simulink model "Project"  (R2021b)
settings: Solver=VariableStepAuto  StartTime=0.0  StopTime=0.02  RelTol=1e-3
model workspace (MAT data in the model file):
  a0 = [1 1 1 1 1 1 1 1 1 1]
undefined symbols (not defined in the file or in its folder): magnitude
libraries: dspstat3 x7, commrflib2 x3, commfilt2 x1
settings Model: Creator=davit  LastModifiedBy=ludovicomazzi
settings SolverCC: AlgebraicLoopSolver=TrustRegion
settings DebuggingCC: SFMachineParentedDataDiag=warning

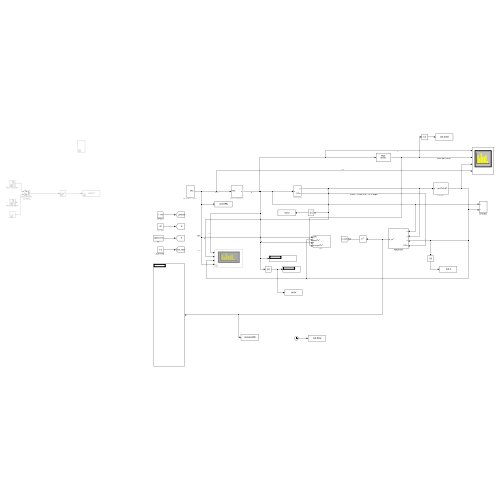
[thumbnail: Simulink's stored preview of the top-level diagram]
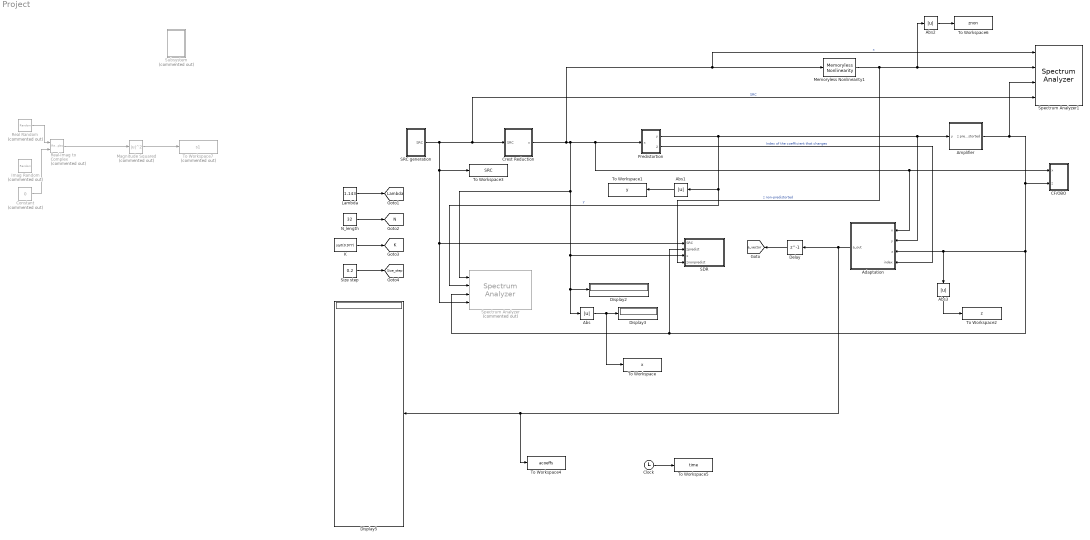
== system Project ==
  Abs{,1..3} (4 alike) : Abs
  Adaptation : Subsystem
  Amplifier : Subsystem
  CF/OBO : Subsystem
  Clock : Clock
  Constant : Constant  Commented=on  Value=0
  Crest Reduction : Subsystem
  Delay : Delay  DelayLength=1
  Display2 : Display
  Display3 : Display
  Display5 : Display
  Imag Random : RandomNumber  Commented=on  Seed=2  SampleTime=1e-7
  K : Constant  Value=sqrt(0.977)
  Lambda : Constant  Value=1.143
  Magnitude Squared : Math  Commented=on  Operator=magnitude^2  SaturateOnIntegerOverflow=on
  Memoryless Nonlinearity1 : commrflib2/Memoryless Nonlinearity  model_select=Rapp model  linGaindB=0  GindB=0  iip3=30  am2pm=10  LPwrLimAMPM=10  UPwrLimAMPM=inf  amam=[2.1587 1.1517]  ampm=[4.0033 9.1040]  x=[8.1081 1.5413 6.5202 -0.0718]  y=[4.6645 2.0965 10.88 -0.003]  p=2.5  GoutdB=0  vsat=1
      settings: SourceProductBaseCode=CM
  N_length : Constant  Value=32
  Predistortion : Subsystem
  Real Random : RandomNumber  Commented=on  Seed=1  SampleTime=1e-7
  Real-Imag to Complex : RealImagToComplex  Commented=on
  SDR : Subsystem
  SRC generation : Subsystem
  Size step : Constant  Value=0.2
  Spectrum Analyzer : SpectrumAnalyzer  Commented=on  NumInputPorts=4
  Spectrum Analyzer1 : SpectrumAnalyzer  NumInputPorts=4
  Subsystem : Subsystem  Commented=on
  To Workspace : ToWorkspace  VariableName=x  SampleTime=-1
      settings: Save2DSignal=2-D array (concatenate along first dimension)
  To Workspace1 : ToWorkspace  VariableName=y  SampleTime=-1
      settings: Save2DSignal=2-D array (concatenate along first dimension)
  To Workspace2 : ToWorkspace  VariableName=z  SampleTime=-1
      settings: Save2DSignal=2-D array (concatenate along first dimension)
  To Workspace3 : ToWorkspace  VariableName=SRC  SampleTime=-1
  To Workspace4 : ToWorkspace  VariableName=acoeffs  SampleTime=-1
      settings: Save2DSignal=2-D array (concatenate along first dimension)
  To Workspace5 : ToWorkspace  VariableName=time  SampleTime=-1
      settings: Save2DSignal=2-D array (concatenate along first dimension)
  To Workspace6 : ToWorkspace  VariableName=znon  SampleTime=-1
      settings: Save2DSignal=2-D array (concatenate along first dimension)
  To Workspace7 : ToWorkspace  Commented=on  VariableName=s1  SampleTime=-1
      settings: Save2DSignal=2-D array (concatenate along first dimension)
  tag scope: K=global, Lambda=global, N=global, Size_step=global, a_vector=global
  wires:
  SRC generation/1(SRC) -> To Workspace3/1, SDR/1(SRC), Spectrum Analyzer/4, Crest Reduction/1(SRC), Spectrum Analyzer1/4  "SRC"
  Crest Reduction/1(x) -> Abs/1, Display2/1, SDR/3(x), Spectrum Analyzer/1, Adaptation/1(x), CF/OBO/1(x), Predistortion/1(x), Spectrum Analyzer1/1, Memoryless Nonlinearity1/1  "x"
  Delay/1 -> [a_vector]
  Abs/1 -> To Workspace/1, Display3/1
  Adaptation/1(a_out) -> Delay/1, To Workspace4/1, Display5/1
  Predistortion/1(y) -> Spectrum Analyzer/2, Abs1/1, Amplifier/1(y), Adaptation/2(y)  "y"
  Predistortion/2(index) -> Adaptation/4(index)  "Index of the coefficient that changes"
  Abs1/1 -> To Workspace1/1
  Lambda/1 -> [Lambda]
  N_length/1 -> [N]
  K/1 -> [K]
  Size step/1 -> [Size_step]
  Clock/1 -> To Workspace5/1
  Memoryless Nonlinearity1/1 -> Spectrum Analyzer1/2, Abs2/1, SDR/4(znonpredist)  "z non-predistorted"
  Abs2/1 -> To Workspace6/1
  Abs3/1 -> To Workspace2/1
  Amplifier/1(z predistorted) -> Spectrum Analyzer1/3, SDR/2(zpredist), Spectrum Analyzer/3, Abs3/1, Adaptation/3(z), CF/OBO/2(z)
  Magnitude Squared/1 -> To Workspace7/1
  Real-Imag to Complex/1 -> Magnitude Squared/1
  Real Random/1 -> Real-Imag to Complex/1
  Constant/1 -> Real-Imag to Complex/2

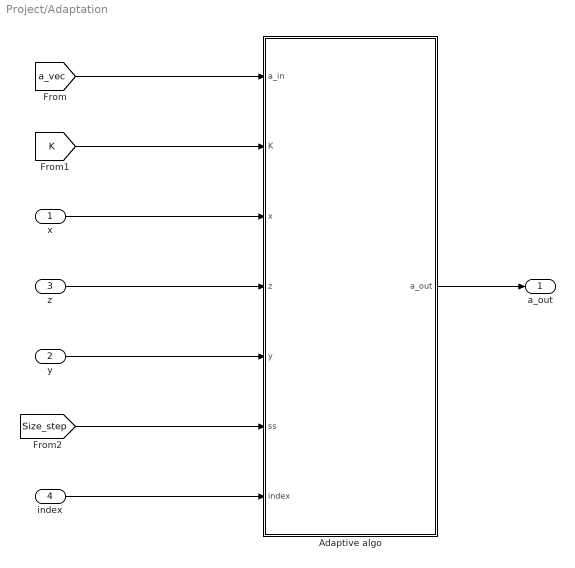
== system Project/Adaptation ==
  x : Inport
  y : Inport  Port=2
  z : Inport  Port=3
  index : Inport  Port=4
  Adaptive algo : MATLAB Function  TreatAsAtomicUnit=on
  a_out : Outport
  wires:
  y/1 -> Adaptive algo/5(y)
  index/1 -> Adaptive algo/7(index)
  z/1 -> Adaptive algo/4(z)
  Adaptive algo/1(a_out) -> a_out/1
  x/1 -> Adaptive algo/3(x)
  [K] -> Adaptive algo/2(K)
  [Size_step] -> Adaptive algo/6(ss)
  [a_vec] -> Adaptive algo/1(a_in)

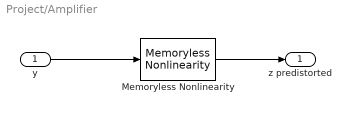
== system Project/Amplifier ==
  y : Inport
  Memoryless Nonlinearity : commrflib2/Memoryless Nonlinearity  model_select=Rapp model  linGaindB=0  GindB=0  iip3=30  am2pm=10  LPwrLimAMPM=10  UPwrLimAMPM=inf  amam=[2.1587 1.1517]  ampm=[4.0033 9.1040]  x=[8.1081 1.5413 6.5202 -0.0718]  y=[4.6645 2.0965 10.88 -0.003]  p=1.5  GoutdB=0  vsat=1
      settings: SourceProductBaseCode=CM
  z predistorted : Outport
  wires:
  Memoryless Nonlinearity/1 -> z predistorted/1
  y/1 -> Memoryless Nonlinearity/1

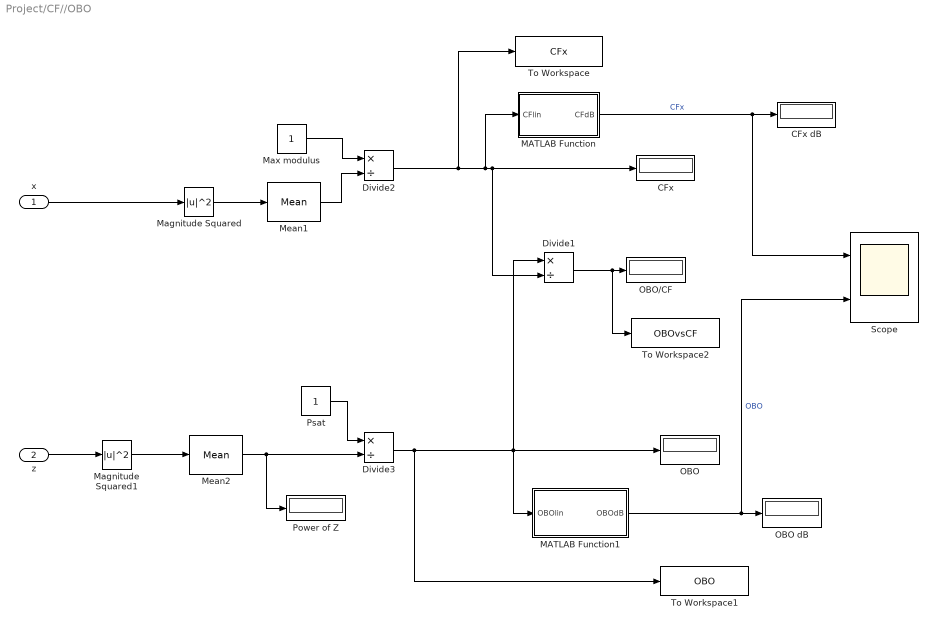
== system Project/CF//OBO ==
  x : Inport
  z : Inport  Port=2
  " CFx" : Display
  " CFx dB" : Display
  " OBO" : Display
  " OBO dB" : Display
  " OBO/CF" : Display
  " Power of Z" : Display
  Divide1 : Product  Inputs=*/
  Divide2 : Product  Inputs=*/
  Divide3 : Product  Inputs=*/
  MATLAB Function : MATLAB Function  TreatAsAtomicUnit=on
  MATLAB Function1 : MATLAB Function  TreatAsAtomicUnit=on
  Magnitude Squared : Math  Operator=magnitude^2  SaturateOnIntegerOverflow=on
  Magnitude Squared1 : Math  Operator=magnitude^2  SaturateOnIntegerOverflow=on
  Max modulus : Constant
  Mean1 : dspstat3/Mean  run=on  reset_popup=None  directionMode=Each column  dimension=1  roiEnable=off  roiType=Rectangles  roiPortion=Entire ROI  roiOutput=Individual statistics for each ROI  roiFlag=off  roundingMode=Nearest  overflowMode=off  outputDataTypeStr=Inherit: Same as accumulator  outputMin=[]  outputMax=[]  outputLastDataTypeStr=Inherit: Same as accumulator
  Mean2 : dspstat3/Mean  run=on  reset_popup=None  directionMode=Each column  dimension=1  roiEnable=off  roiType=Rectangles  roiPortion=Entire ROI  roiOutput=Individual statistics for each ROI  roiFlag=off  roundingMode=Nearest  overflowMode=off  outputDataTypeStr=Inherit: Same as accumulator  outputMin=[]  outputMax=[]  outputLastDataTypeStr=Inherit: Same as accumulator
  Psat : Constant
  Scope : Scope  NumInputPorts=2
  To Workspace : ToWorkspace  VariableName=CFx  SampleTime=-1
      settings: Save2DSignal=2-D array (concatenate along first dimension)
  To Workspace1 : ToWorkspace  VariableName=OBO  SampleTime=-1
      settings: Save2DSignal=2-D array (concatenate along first dimension)
  To Workspace2 : ToWorkspace  VariableName=OBOvsCF  SampleTime=-1
      settings: Save2DSignal=2-D array (concatenate along first dimension)
  wires:
  MATLAB Function/1(CFdB) -> Scope/1, " CFx dB"/1  "CFx"
  Divide1/1 -> To Workspace2/1, " OBO/CF"/1
  MATLAB Function1/1(OBOdB) -> Scope/2, " OBO dB"/1  "OBO"
  Magnitude Squared/1 -> Mean1/1
  x/1 -> Magnitude Squared/1
  Mean1/1 -> Divide2/2
  Max modulus/1 -> Divide2/1
  z/1 -> Magnitude Squared1/1
  Magnitude Squared1/1 -> Mean2/1
  Mean2/1 -> " Power of Z"/1, Divide3/2
  Divide3/1 -> MATLAB Function1/1(OBOlin), " OBO"/1, Divide1/1, To Workspace1/1
  Divide2/1 -> " CFx"/1, Divide1/2, MATLAB Function/1(CFlin), To Workspace/1
  Psat/1 -> Divide3/1

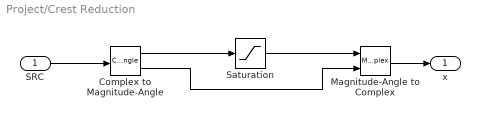
== system Project/Crest Reduction ==
  SRC : Inport
  Complex to Magnitude-Angle : ComplexToMagnitudeAngle
  Magnitude-Angle to Complex : MagnitudeAngleToComplex
  Saturation : Saturate  UpperLimit=1  LowerLimit=0  RndMeth=Nearest
  x : Outport
  wires:
  Magnitude-Angle to Complex/1 -> x/1
  Saturation/1 -> Magnitude-Angle to Complex/1
  Complex to Magnitude-Angle/2 -> Magnitude-Angle to Complex/2
  Complex to Magnitude-Angle/1 -> Saturation/1
  SRC/1 -> Complex to Magnitude-Angle/1

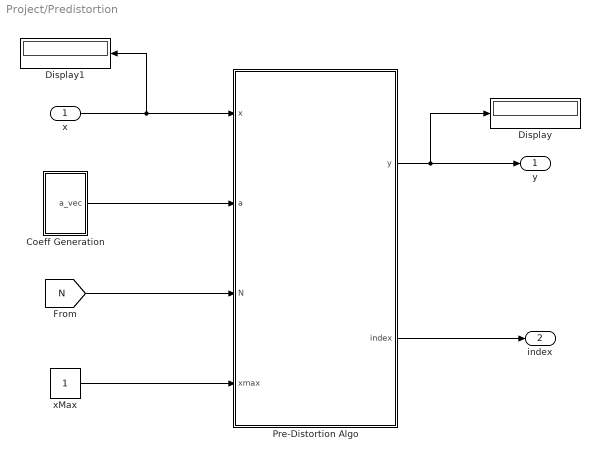
== system Project/Predistortion ==
  x : Inport
  Coeff Generation : Subsystem
  Display : Display
  Display1 : Display
  Pre-Distortion Algo : MATLAB Function  TreatAsAtomicUnit=on
  xMax : Constant
  y : Outport
  index : Outport  Port=2
  wires:
  [N] -> Pre-Distortion Algo/3(N)
  Pre-Distortion Algo/2(index) -> index/1
  Pre-Distortion Algo/1(y) -> Display/1, y/1
  x/1 -> Display1/1, Pre-Distortion Algo/1(x)
  xMax/1 -> Pre-Distortion Algo/4(xmax)
  Coeff Generation/1(a_vec) -> Pre-Distortion Algo/2(a)

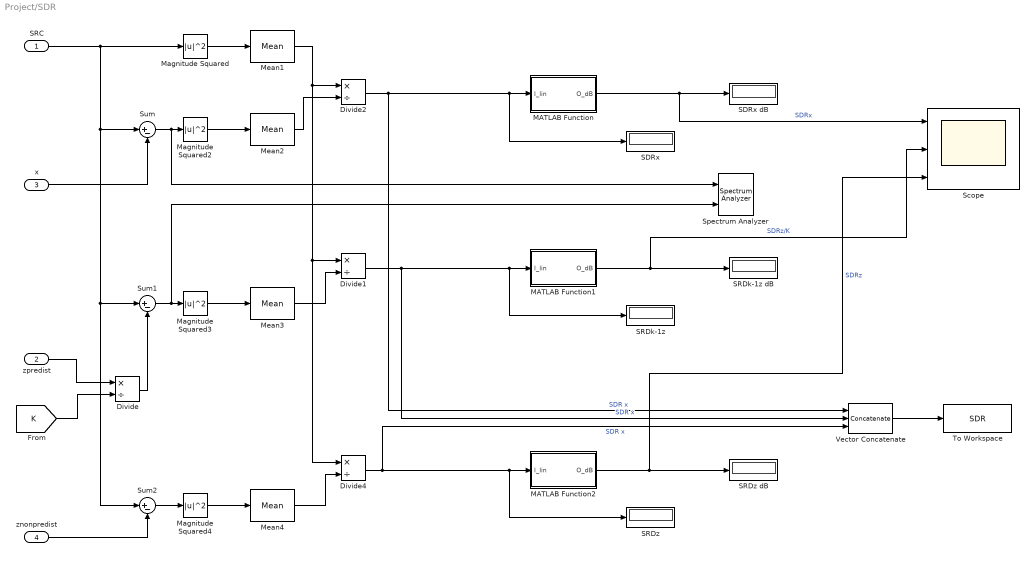
== system Project/SDR ==
  SRC : Inport
  zpredist : Inport  Port=2
  x : Inport  Port=3
  znonpredist : Inport  Port=4
  " SDRx" : Display
  " SDRx dB" : Display
  " SRDk-1z" : Display
  " SRDk-1z dB" : Display
  " SRDz" : Display
  Divide{,1..2,4} (4 alike) : Product  Inputs=*/
  MATLAB Function : MATLAB Function  TreatAsAtomicUnit=on
  MATLAB Function1 : MATLAB Function  TreatAsAtomicUnit=on
  MATLAB Function2 : MATLAB Function  TreatAsAtomicUnit=on
  Magnitude Squared{,2..4} (4 alike) : Math  Operator=magnitude^2  SaturateOnIntegerOverflow=on
  Mean{1..4} (4 alike) : dspstat3/Mean  run=on  reset_popup=None  directionMode=Each column  dimension=1  roiEnable=off  roiType=Rectangles  roiPortion=Entire ROI  roiOutput=Individual statistics for each ROI  roiFlag=off  roundingMode=Nearest  overflowMode=off  outputDataTypeStr=Inherit: Same as accumulator  outputMin=[]  outputMax=[]  outputLastDataTypeStr=Inherit: Same as accumulator
  SRDz dB : Display
  Scope : Scope  NumInputPorts=3
  Spectrum Analyzer : SpectrumAnalyzer  NumInputPorts=2
  Sum : Sum  Inputs=|+-
  Sum1 : Sum  Inputs=|+-
  Sum2 : Sum  Inputs=|+-
  To Workspace : ToWorkspace  VariableName=SDR  SampleTime=-1
      settings: Save2DSignal=2-D array (concatenate along first dimension)
  Vector Concatenate : Concatenate  NumInputs=3
  wires:
  Magnitude Squared/1 -> Mean1/1
  x/1 -> Sum/2
  Sum/1 -> Spectrum Analyzer/1, Magnitude Squared2/1
  Mean2/1 -> Divide2/2
  Magnitude Squared2/1 -> Mean2/1
  Sum1/1 -> Spectrum Analyzer/2, Magnitude Squared3/1
  Mean3/1 -> Divide1/2
  Magnitude Squared3/1 -> Mean3/1
  Sum2/1 -> Magnitude Squared4/1
  SRC/1 -> Magnitude Squared/1, Sum/1, Sum1/1, Sum2/1
  Mean4/1 -> Divide4/2
  Magnitude Squared4/1 -> Mean4/1
  Mean1/1 -> Divide4/1, Divide1/1, Divide2/1
  [K] -> Divide/2
  Divide/1 -> Sum1/2
  znonpredist/1 -> Sum2/2
  zpredist/1 -> Divide/1
  MATLAB Function/1(O_dB) -> Scope/1, " SDRx dB"/1  "SDRx"
  MATLAB Function1/1(O_dB) -> " SRDk-1z dB"/1, Scope/2  "SDRz/K"
  MATLAB Function2/1(O_dB) -> SRDz dB/1, Scope/3  "SDRz"
  Divide2/1 -> " SDRx"/1, MATLAB Function/1(I_lin), Vector Concatenate/1  "SDR x"
  Divide4/1 -> MATLAB Function2/1(I_lin), " SRDz"/1, Vector Concatenate/3  "SDR x"
  Divide1/1 -> MATLAB Function1/1(I_lin), " SRDk-1z"/1, Vector Concatenate/2  "SDR x"
  Vector Concatenate/1 -> To Workspace/1

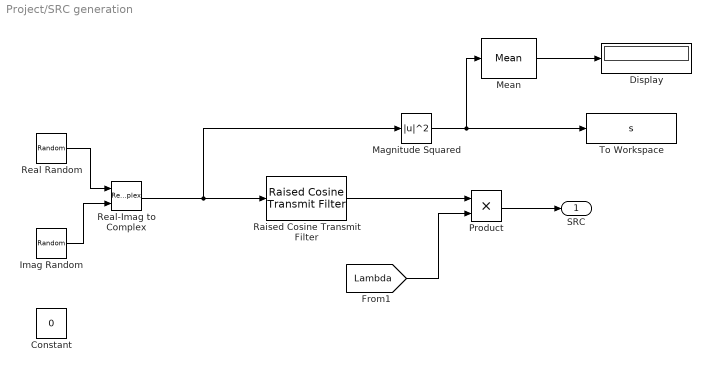
== system Project/SRC generation ==
  Constant : Constant  Value=0
  Display : Display
  Imag Random : RandomNumber  Variance=1/2  Seed=2  SampleTime=1e-7
  Magnitude Squared : Math  Operator=magnitude^2  SaturateOnIntegerOverflow=on
  Mean : dspstat3/Mean  run=on  reset_popup=None  directionMode=Entire input  dimension=1  roiEnable=off  roiType=Rectangles  roiPortion=Entire ROI  roiOutput=Individual statistics for each ROI  roiFlag=off  roundingMode=Nearest  overflowMode=off  outputDataTypeStr=Inherit: Same as accumulator  outputMin=[]  outputMax=[]  outputLastDataTypeStr=Inherit: Same as accumulator
  Product : Product
  Raised Cosine Transmit Filter : commfilt2/Raised Cosine Transmit Filter  filtType=Square root  R=0.2  filtSpan=80  N=8  filterGain=1  RateOptions=Allow multirate processing  framing=Mute  checkCoeff=off  variableName=rcTxFilt  checkGain=Normalized  sampMode=Mute  saveAsFlag=0  currentFiltSpan=10  D=5  launchFVT=on  roundingMode=Floor  overflowMode=off  coeffDataTypeStr=Inherit: Same word length as input  coeffMin=[]  coeffMax=[]  coeffLastDataTypeStr=Inherit: Same word length as input  outputDataTypeStr=Inherit: Same as accumulator  outputMin=[]  outputMax=[]  outputLastDataTypeStr=Inherit: Same as accumulator
  Real Random : RandomNumber  Variance=1/2  Seed=1  SampleTime=1e-7
  Real-Imag to Complex : RealImagToComplex
  To Workspace : ToWorkspace  VariableName=s  SampleTime=-1
      settings: Save2DSignal=2-D array (concatenate along first dimension)
  SRC : Outport
  wires:
  [Lambda] -> Product/2
  Product/1 -> SRC/1
  Magnitude Squared/1 -> Mean/1, To Workspace/1
  Raised Cosine Transmit Filter/1 -> Product/1
  Real-Imag to Complex/1 -> Magnitude Squared/1, Raised Cosine Transmit Filter/1
  Real Random/1 -> Real-Imag to Complex/1
  Mean/1 -> Display/1
  Imag Random/1 -> Real-Imag to Complex/2

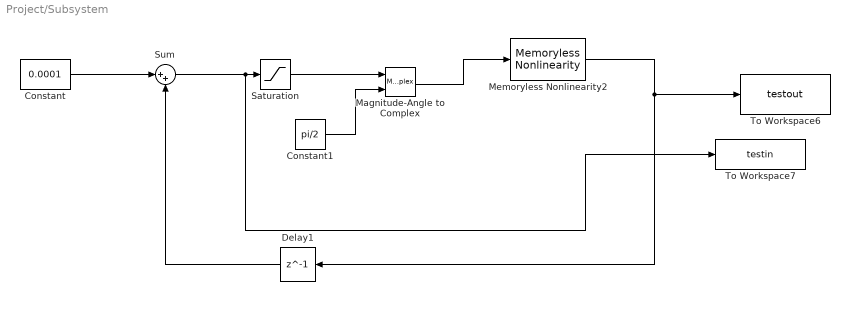
== system Project/Subsystem ==
  Constant : Constant  Value=0.0001
  Constant1 : Constant  Value=pi/2
  Delay1 : Delay  DelayLength=1
  Magnitude-Angle to Complex : MagnitudeAngleToComplex
  Memoryless Nonlinearity2 : commrflib2/Memoryless Nonlinearity  model_select=Rapp model  linGaindB=0  GindB=0  iip3=30  am2pm=10  LPwrLimAMPM=10  UPwrLimAMPM=inf  amam=[2.1587 1.1517]  ampm=[4.0033 9.1040]  x=[8.1081 1.5413 6.5202 -0.0718]  y=[4.6645 2.0965 10.88 -0.003]  p=3  GoutdB=0  vsat=1
      settings: SourceProductBaseCode=CM
  Saturation : Saturate  UpperLimit=1  LowerLimit=0
  Sum : Sum  Inputs=|++
  To Workspace6 : ToWorkspace  VariableName=testout  SampleTime=-1
      settings: Save2DSignal=2-D array (concatenate along first dimension)
  To Workspace7 : ToWorkspace  VariableName=testin  SaveFormat=Timeseries  SampleTime=-1
  wires:
  Delay1/1 -> Sum/2
  Constant/1 -> Sum/1
  Constant1/1 -> Magnitude-Angle to Complex/2
  Sum/1 -> To Workspace7/1, Saturation/1
  Memoryless Nonlinearity2/1 -> Delay1/1, To Workspace6/1
  Saturation/1 -> Magnitude-Angle to Complex/1
  Magnitude-Angle to Complex/1 -> Memoryless Nonlinearity2/1

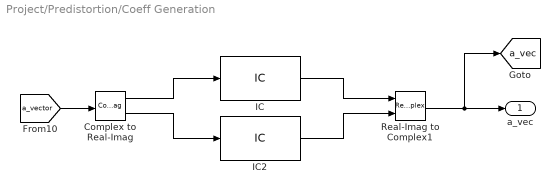
== system Project/Predistortion/Coeff Generation ==
  Complex to Real-Imag : ComplexToRealImag
  IC : InitialCondition  Value=ones(1,33)
  IC2 : InitialCondition  Value=zeros(1,33)
  Real-Imag to Complex1 : RealImagToComplex
  a_vec : Outport
  tag scope: a_vec=global
  wires:
  Complex to Real-Imag/1 -> IC/1
  Complex to Real-Imag/2 -> IC2/1
  [a_vector] -> Complex to Real-Imag/1
  IC/1 -> Real-Imag to Complex1/1
  IC2/1 -> Real-Imag to Complex1/2
  Real-Imag to Complex1/1 -> [a_vec], a_vec/1

== matlab function Project/Adaptation/Adaptive algo ==
  data: a_in input; a_out output; K input; x input; z input; y input; ss input; index input
function a_out = Adaptation(a_in, K, x, z, y, ss, index)

% Adaptive algorithm
a_out = a_in; 
a_out(index) = abs(a_in(index) - ss*(z-K*x) * ((conj(z) / conj(y)) * conj(x))); 

end

== matlab function Project/SDR/MATLAB Function ==
  data: I_lin input; O_dB output
function O_dB = lintodb(I_lin)

O_dB = 10.*log10(I_lin);

== matlab function Project/SDR/MATLAB Function1 ==
  data: I_lin input; O_dB output
function O_dB = lintodb(I_lin)

O_dB = 10.*log10(I_lin);

== matlab function Project/Predistortion/Pre-Distortion Algo ==
  data: x input; y output; a input; N input; xmax input; index output
function [y,index]  = PreDist(x, a, N, xmax)

delta = abs(xmax)/(2*N);

I = [2*delta:2*delta:xmax 100];
n = 1:(N+1);
n = n(abs(x)<I);
n = n(1);
index = n;

P_x = ((abs(x) - (2*n+1)*delta) * (a(min(n+1,N+1)) - a(n)) / (2*delta)) + ((a(min(n+1,N+1)) + a(n)) / 2);
y = complex(x*P_x);

end

== matlab function Project/CF//OBO/MATLAB Function ==
  data: CFlin input; CFdB output
function CFdB = lintodb(CFlin)
CFdB = 10.*log10(CFlin);

== matlab function Project/CF//OBO/MATLAB Function1 ==
  data: OBOlin input; OBOdB output
function OBOdB = lintodb(OBOlin)
OBOdB = 10*log10(OBOlin);

== matlab function Project/SDR/MATLAB Function2 ==
  data: I_lin input; O_dB output
function O_dB = lintodb(I_lin)

O_dB = 10.*log10(I_lin);
